simulink model "TVC_FSFB_model"  (R2024b)
settings: Solver=ode8  StartTime=0.0  StopTime=140  FixedStep=0.0001  RelTol=1e-3
values from neighbouring files (symbols this model uses):
  A_plant = double(A_plant_raw)    [LQR_Heavy_STeVe.m]    (also in control_system_analysis.m = [-Z_alpha/V, 1, 0; M_alpha, M_q, 0; 0, 1, 0]; mid_loop_controller.m = A_airframe; robustness_analysis.m = [-Z_alpha/V,  1,   0)
  B_plant = double(B_plant_raw)    [LQR_Heavy_STeVe.m]    (also in control_system_analysis.m = [-Z_delta/V; M_delta; 0]; mid_loop_controller.m = B_airframe; robustness_analysis.m = [-Z_delta/V)
  C_plant = double(eye(3))    [LQR_Heavy_STeVe.m]    (also in mid_loop_controller.m = [eye(3))
  D_plant = double(zeros(3,1))    [LQR_Heavy_STeVe.m]    (also in mid_loop_controller.m = [zeros(3,1))
  K_lqr = lqr(A, B, Q, R)    [LQR_Heavy_STeVe.m]    (also in mid_loop_controller.m = K; robustness_analysis.m = lqr(A_ol, B_ol, Q, R))
libraries: simulink_extras x4, aerolibactuator x2
settings Model: Creator=jonno  LastModifiedBy=jonno

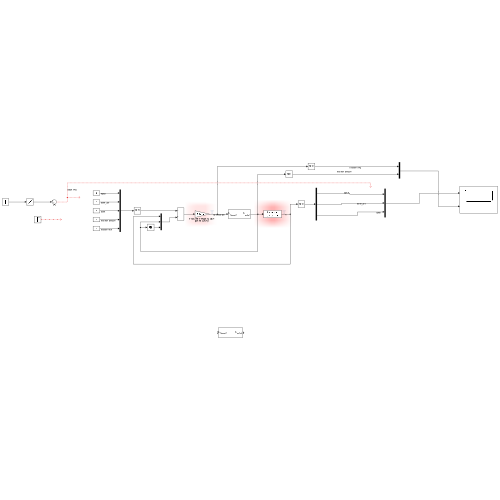
[thumbnail: Simulink's stored preview of the top-level diagram]
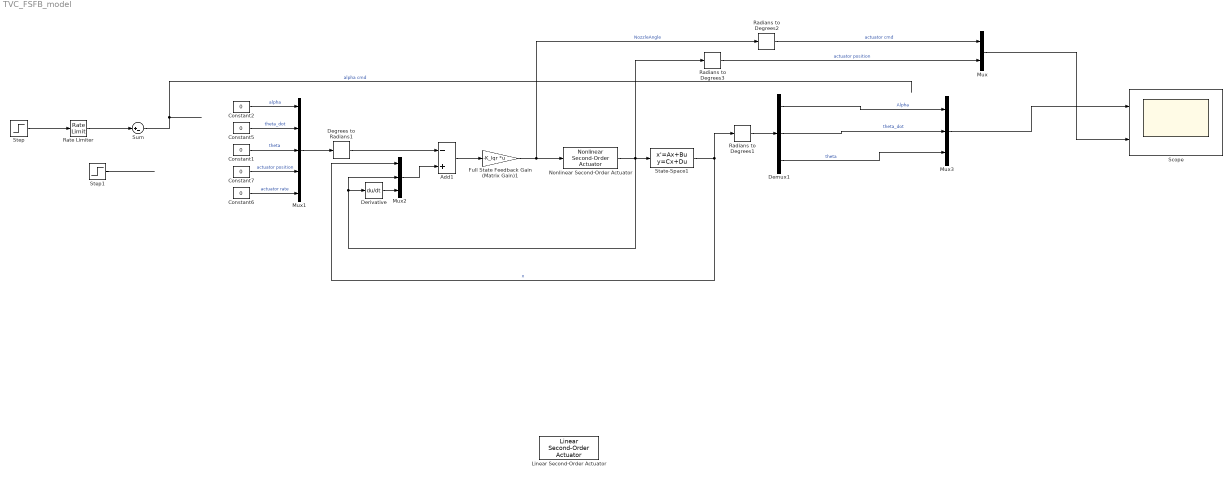
== system TVC_FSFB_model ==
  Add1 : Sum  Inputs=-+
  Constant{1..2,5..7} (5 alike) : Constant  Value=0
  Degrees to Radians1 : simulink_extras/Transformations/Degrees to Radians
  Demux1 : Demux  Outputs=3
  Derivative : Derivative
  Full State Feedback Gain (Matrix Gain)1 : Gain  Gain=-K_lqr  Multiplication=Matrix(K*u)
  Linear Second-Order Actuator : aerolibactuator/Linear Second-Order Actuator  wn_fin=62  z_fin=0.5858  fin_act_0=0  fin_act_vel=0
  Mux : Mux  Inputs=2
  Mux1 : Mux  Inputs=5
  Mux2 : Mux  Inputs=3
  Mux3 : Mux  Inputs=3
  Nonlinear Second-Order Actuator : aerolibactuator/Nonlinear Second-Order Actuator  wn_fin=62  z_fin=0.545  fin_max=5*pi/180  fin_min=-5*pi/180  fin_maxrate=500*pi/180  fin_act_0=0  fin_act_vel=0
  Radians to Degrees1 : simulink_extras/Transformations/Radians to Degrees
  Radians to Degrees2 : simulink_extras/Transformations/Radians to Degrees
  Radians to Degrees3 : simulink_extras/Transformations/Radians to Degrees
  Rate Limiter : RateLimiter  RisingSlewLimit=0.1  FallingSlewLimit=-0.1  SampleTimeMode=inherited
  Scope : Scope  NumInputPorts=2
  State-Space1 : StateSpace  A=A_plant  B=B_plant  C=C_plant  D=D_plant  InitialCondition=[2*pi/180; 0; 0]
  Step : Step  After=0.1  SampleTime=0
  Step1 : Step  Time=4  After=10*pi/180  SampleTime=0
  Sum : Sum  Inputs=|+-
  wires:
  Demux1/2 -> Mux3/2  "theta_dot"
  Degrees to Radians1/1 -> Add1/1
  Mux1/1 -> Degrees to Radians1/1
  Constant7/1 -> Mux1/4  "actuator position"
  Constant6/1 -> Mux1/5  "actuator rate"
  Add1/1 -> Full State Feedback Gain (Matrix Gain)1/1
  Full State Feedback Gain (Matrix Gain)1/1 -> Nonlinear Second-Order Actuator/1, Radians to Degrees2/1  "NozzleAngle"
  Constant5/1 -> Mux1/2  "theta_dot"
  State-Space1/1 -> Mux2/1, Radians to Degrees1/1  "x"
  Demux1/1 -> Mux3/1  "Alpha"
  Demux1/3 -> Mux3/3  "theta"
  Radians to Degrees3/1 -> Mux/2  "actuator position"
  Radians to Degrees1/1 -> Demux1/1
  Mux2/1 -> Add1/2
  Nonlinear Second-Order Actuator/1 -> Mux2/2, Derivative/1, Radians to Degrees3/1, State-Space1/1
  Radians to Degrees2/1 -> Mux/1  "actuator cmd"
  Derivative/1 -> Mux2/3
  Step/1 -> Rate Limiter/1
  Mux/1 -> Scope/2
  Step1/1 -> ?
  Constant2/1 -> Mux1/1  "alpha"
  Mux3/1 -> Scope/1
  Sum/1 -> ?  "alpha cmd"
  Constant1/1 -> Mux1/3  "theta"
  Rate Limiter/1 -> Sum/1
